simulink library "bcm"  (R2021b)
settings: Solver=VariableStepAuto  StartTime=0.0  StopTime=10.0  RelTol=1e-3
undefined symbols (not defined in the file or in its folder): ENUM_ANTITHEFT_ALARM, ENUM_ANTITHEFT_ARM, ENUM_ANTITHEFT_DISARM, ENUM_ANTITHEFT_WAIT, ENUM_GEARPOSNTOCAN_P, ENUM_PDKEYRAWLULOCK_INUNLOCK, ENUM_PDKEYRAWPS_INPS, ENUM_POWERSTA_ON, ENUM_POWERSTA_READY, ENUM_POWERSTA_STANDBY, FALSE, KBCM_ALMBrightnessDark_enum, KBCM_AmbBlue_enum, KBCM_AmbBreathT_ms, KBCM_AmbGreen_enum, KBCM_AmbRed_enum, KBCM_Antitheft_enum_ovrdflg, KBCM_Antitheft_enum_ovrdval, KBCM_APMDoorCtrlSta_flg_ovrdflg, KBCM_APMDoorCtrlSta_flg_ovrdval, KBCM_DelayTSW_flg, KBCM_DiagFLTC_mA, KBCM_DiagFMHT_s, KBCM_DiagFRTC_mA, KBCM_DiagRLTC_mA, KBCM_DiagRRTC_mA, KBCM_DrAPMRetryTimes_cnt, KBCM_DrOpenWdwOT_s, KBCM_DrOpenWdwReady_s, KBCM_ESSOffT_ms, KBCM_ESSOnT_ms, KBCM_IVIRstHoldT_ms, KBCM_IVIRstTriggerT_ms, KBCM_ONDelayT_ms, KBCM_ReDetectT_K, KBCM_RmLampKeep_min, KBCM_RmLpKeyInT_s, KBCM_RmLpKeyMissT_s, KBCM_SlpDebounceTime_s, KBCM_SPTGDetectT_sec, KBCM_SPTGLeave_flg, KBCM_SPTGLeftBound_cm, KBCM_SPTGLeftBoundOut_cm, KBCM_SPTGLowerBound_cm, KBCM_SPTGLowerBoundOut_cm, KBCM_SPTGRightBound_cm, KBCM_SPTGRightBoundOut_cm, KBCM_SPTGTOut_K, KBCM_SPTGUpperBound_cm, KBCM_SPTGUpperBoundOut_cm, KBCM_SPTGWaitDKC_sec, KBCM_TrunSWKeepTime3_s, KBCM_TrunSWKeepTime5_s, KBCM_TrunSWKeepTime7_s, KBCM_USSDis_cm, KBCM_USSFilterT_K, KBCM_WaitAPMPwr_K, KBCM_WdwManualDetT_s, MIN2SEC, TRUE ... (+1)
libraries: simulink x151, hcu_lib x5
(part 6 of 8)

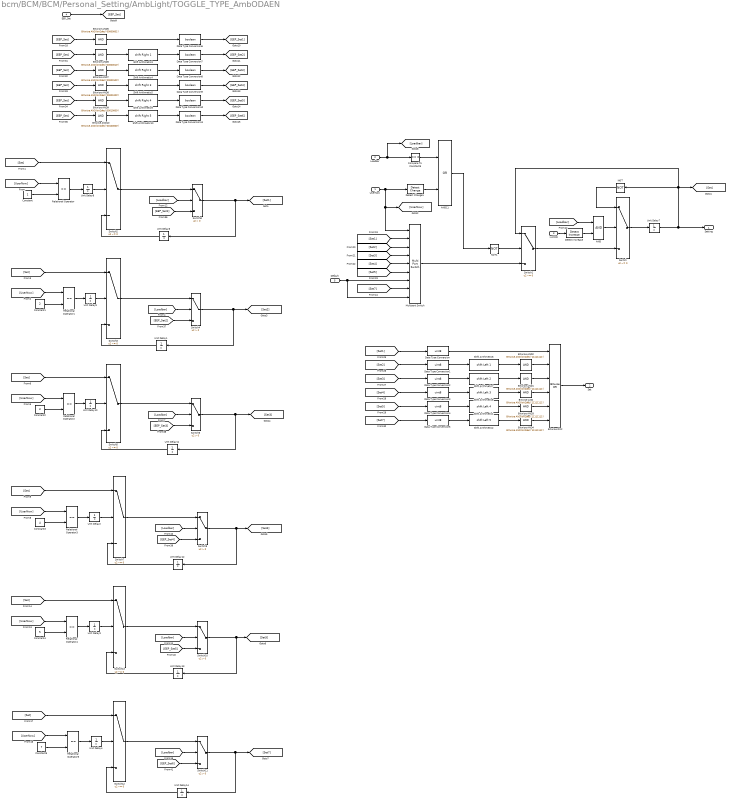
== system bcm/BCM/BCM/Personal_Setting/AmbLight/TOGGLE_TYPE_AmbODAEN ==
  UserNow : Inport
  Loadbar : Inport  Port=2
  iviCMD : Inport  Port=3
  EEP_Set : Inport  Port=4
  Default : Inport  Port=5
  AND : Logic  AllPortsSameDT=off  OutDataTypeStr=boolean
  AND11 : Logic  Operator=OR  AllPortsSameDT=off  OutDataTypeStr=boolean
  Bitwise AND{,1..4} (5 alike) : simulink/Logic and Bit Operations/Bitwise Operator  logicop=AND  UseBitMask=on  BitMask=bin2dec('11111111')  BitMaskRealWorld=Stored Integer
  Bitwise AND10 : simulink/Logic and Bit Operations/Bitwise Operator  logicop=AND  UseBitMask=on  BitMask=bin2dec('00100000')  BitMaskRealWorld=Stored Integer
  Bitwise AND5 : simulink/Logic and Bit Operations/Bitwise Operator  logicop=AND  UseBitMask=on  BitMask=bin2dec('00000001')  BitMaskRealWorld=Stored Integer
  Bitwise AND6 : simulink/Logic and Bit Operations/Bitwise Operator  logicop=AND  UseBitMask=on  BitMask=bin2dec('00000010')  BitMaskRealWorld=Stored Integer
  Bitwise AND7 : simulink/Logic and Bit Operations/Bitwise Operator  logicop=AND  UseBitMask=on  BitMask=bin2dec('00000100')  BitMaskRealWorld=Stored Integer
  Bitwise AND8 : simulink/Logic and Bit Operations/Bitwise Operator  logicop=AND  UseBitMask=on  BitMask=bin2dec('00001000')  BitMaskRealWorld=Stored Integer
  Bitwise AND9 : simulink/Logic and Bit Operations/Bitwise Operator  logicop=AND  UseBitMask=on  BitMask=bin2dec('00010000')  BitMaskRealWorld=Stored Integer
  Bitwise OR2 : simulink/Logic and Bit Operations/Bitwise Operator  logicop=OR  UseBitMask=off  NumInputPorts=6  BitMask=bin2dec('00000000000000000000')  BitMaskRealWorld=Stored Integer
  Compare To Constant5 : simulink/Logic and Bit Operations/Compare To Constant  relop===  const=0  OutDataTypeStr=boolean
  Constant : Constant  OutDataTypeStr=uint8
  Constant1 : Constant  Value=2  OutDataTypeStr=uint8
  Constant2 : Constant  Value=3  OutDataTypeStr=uint8
  Constant3 : Constant  Value=4  OutDataTypeStr=uint8
  Constant4 : Constant  Value=5  OutDataTypeStr=uint8
  Constant5 : Constant  Value=7  OutDataTypeStr=uint8
  Data Type Conversion{,1..5} (6 alike) : DataTypeConversion  OutDataTypeStr=uint8
  Data Type Conversion{6..11} (6 alike) : DataTypeConversion  OutDataTypeStr=boolean
  Detect Change1 : simulink/Logic and Bit Operations/Detect Change  vinit=0  OutDataTypeStr=boolean
  Detect Increase : simulink/Logic and Bit Operations/Detect Increase  vinit=0.0  OutDataTypeStr=boolean
  Multiport Switch : MultiPortSwitch  Inputs=7  DataPortForDefault=Additional data port  DiagnosticForDefault=None
  NOT : Logic  Operator=NOT  IconShape=distinctive  AllPortsSameDT=off  OutDataTypeStr=boolean
  NOT1 : Logic  Operator=NOT  IconShape=distinctive  AllPortsSameDT=off  OutDataTypeStr=boolean
  Relational Operator{,1..5} (6 alike) : RelationalOperator  Operator===  OutDataTypeStr=boolean  RndMeth=Simplest
  Shift Arithmetic1 : ArithShift  BitShiftNumber=4  BitShiftDirection=Left
  Shift Arithmetic10 : ArithShift  BitShiftNumber=5  BitShiftDirection=Right
  Shift Arithmetic2 : ArithShift  BitShiftNumber=5  BitShiftDirection=Left
  Shift Arithmetic3 : ArithShift  BitShiftNumber=1  BitShiftDirection=Right
  Shift Arithmetic4 : ArithShift  BitShiftNumber=2  BitShiftDirection=Right
  Shift Arithmetic5 : ArithShift  BitShiftNumber=3  BitShiftDirection=Right
  Shift Arithmetic6 : ArithShift  BitShiftNumber=1  BitShiftDirection=Left
  Shift Arithmetic7 : ArithShift  BitShiftNumber=2  BitShiftDirection=Left
  Shift Arithmetic8 : ArithShift  BitShiftNumber=3  BitShiftDirection=Left
  Shift Arithmetic9 : ArithShift  BitShiftNumber=4  BitShiftDirection=Right
  Switch{,1..3,5,7,12..13} (8 alike) : Switch  Criteria=u2 ~= 0
  Switch{4,6,8..11} (6 alike) : Switch  Criteria=u2 > Threshold
  Unit Delay{1..4,6..14} (13 alike) : UnitDelay  SampleTime=-1  HasFrameUpgradeWarning=on
  Setting : Outport
  Set : Outport  Port=2
  wires:
  [Loadbar] -> AND/1
  Detect Increase/1 -> AND/2
  AND/1 -> Switch/2
  Unit Delay14/1 -> Switch12/3
  Unit Delay4/1 -> Switch12/2
  Unit Delay13/1 -> Switch13/3
  Unit Delay3/1 -> Switch13/2
  Unit Delay12/1 -> Switch7/3
  Unit Delay2/1 -> Switch7/2
  Unit Delay11/1 -> Switch5/3
  Unit Delay10/1 -> Switch5/2
  Unit Delay9/1 -> Switch3/2
  Unit Delay8/1 -> Switch2/2
  Unit Delay1/1 -> Switch3/3
  Unit Delay6/1 -> Switch2/3
  Relational Operator1/1 -> Unit Delay9/1
  Relational Operator/1 -> Unit Delay8/1
  [EEP_Set6] -> Switch11/3
  [EEP_Set5] -> Switch10/3
  [EEP_Set4] -> Switch9/3
  [EEP_Set3] -> Switch6/3
  [EEP_Set2] -> Switch4/3
  [EEP_Set1] -> Switch8/3
  Data Type Conversion11/1 -> [EEP_Set6]
  Data Type Conversion10/1 -> [EEP_Set5]
  Data Type Conversion9/1 -> [EEP_Set4]
  Data Type Conversion8/1 -> [EEP_Set3]
  Data Type Conversion7/1 -> [EEP_Set2]
  Data Type Conversion6/1 -> [EEP_Set1]
  [EEP_Set] -> Bitwise AND10/1
  [EEP_Set] -> Bitwise AND9/1
  [EEP_Set] -> Bitwise AND8/1
  [EEP_Set] -> Bitwise AND7/1
  [EEP_Set] -> Bitwise AND6/1
  [EEP_Set] -> Bitwise AND5/1
  EEP_Set/1 -> [EEP_Set]
  Shift Arithmetic5/1 -> Data Type Conversion9/1
  Shift Arithmetic9/1 -> Data Type Conversion10/1
  Bitwise AND7/1 -> Shift Arithmetic4/1
  Shift Arithmetic3/1 -> Data Type Conversion7/1
  Bitwise AND5/1 -> Data Type Conversion6/1
  Shift Arithmetic10/1 -> Data Type Conversion11/1
  Shift Arithmetic4/1 -> Data Type Conversion8/1
  Bitwise AND10/1 -> Shift Arithmetic10/1
  Bitwise AND9/1 -> Shift Arithmetic9/1
  Bitwise AND6/1 -> Shift Arithmetic3/1
  Bitwise AND8/1 -> Shift Arithmetic5/1
  Bitwise OR2/1 -> Set/1
  [Set3] -> Data Type Conversion2/1
  Bitwise AND4/1 -> Bitwise OR2/6
  Data Type Conversion1/1 -> Shift Arithmetic6/1
  Bitwise AND/1 -> Bitwise OR2/4
  [Set5] -> Data Type Conversion4/1
  [Set1] -> Data Type Conversion/1
  Data Type Conversion3/1 -> Shift Arithmetic8/1
  [Set2] -> Data Type Conversion1/1
  Data Type Conversion/1 -> Bitwise OR2/1
  [Set7] -> Data Type Conversion5/1
  Shift Arithmetic1/1 -> Bitwise AND3/1
  Shift Arithmetic7/1 -> Bitwise AND1/1
  Data Type Conversion4/1 -> Shift Arithmetic1/1
  Shift Arithmetic6/1 -> Bitwise AND2/1
  Bitwise AND2/1 -> Bitwise OR2/2
  Bitwise AND1/1 -> Bitwise OR2/3
  Bitwise AND3/1 -> Bitwise OR2/5
  Shift Arithmetic2/1 -> Bitwise AND4/1
  Shift Arithmetic8/1 -> Bitwise AND/1
  [Set4] -> Data Type Conversion3/1
  Data Type Conversion5/1 -> Shift Arithmetic2/1
  Data Type Conversion2/1 -> Shift Arithmetic7/1
  Relational Operator5/1 -> Unit Delay4/1
  Relational Operator4/1 -> Unit Delay3/1
  Relational Operator3/1 -> Unit Delay2/1
  Relational Operator2/1 -> Unit Delay10/1
  Unit Delay7/1 -> Switch1/1, [Set], NOT/1, Setting/1
  Switch11/1 -> Unit Delay14/1, [Set7]
  Switch12/1 -> Switch11/1
  Switch10/1 -> Unit Delay13/1, [Set5]
  Switch9/1 -> Unit Delay12/1, [Set4]
  Switch7/1 -> Switch9/1
  Switch5/1 -> Switch6/1
  Switch6/1 -> Unit Delay11/1, [Set3]
  Switch4/1 -> Unit Delay1/1, [Set2]
  Switch3/1 -> Switch4/1
  Switch2/1 -> Switch8/1
  Switch8/1 -> Unit Delay6/1, [Set1]
  Switch/1 -> Unit Delay7/1
  AND11/1 -> NOT1/1
  Compare To Constant5/1 -> AND11/1
  Constant4/1 -> Relational Operator4/2
  [Loadbar] -> Switch8/2
  [Set] -> Switch5/1
  [Loadbar] -> Switch6/2
  [Set] -> Switch7/1
  Constant1/1 -> Relational Operator1/2
  [UserNow] -> Relational Operator4/1
  [Set] -> Switch2/1
  Constant3/1 -> Relational Operator3/2
  [UserNow] -> Relational Operator3/1
  [UserNow] -> Relational Operator2/1
  [Loadbar] -> Switch9/2
  Constant/1 -> Relational Operator/2
  [Set] -> Switch3/1
  [Loadbar] -> Switch11/2
  Constant2/1 -> Relational Operator2/2
  [Loadbar] -> Switch10/2
  [UserNow] -> Relational Operator1/1
  [UserNow] -> Relational Operator/1
  Constant5/1 -> Relational Operator5/2
  [UserNow] -> Relational Operator5/1
  [Set] -> Switch12/1
  [Loadbar] -> Switch4/2
  [Set] -> Switch13/1
  iviCMD/1 -> Detect Increase/1
  NOT/1 -> Switch/1
  UserNow/1 -> Detect Change1/1, [UserNow], Multiport Switch/1
  Switch1/1 -> Switch/3
  Loadbar/1 -> Compare To Constant5/1, [Loadbar]
  Multiport Switch/1 -> Switch1/3
  Detect Change1/1 -> AND11/2
  Switch13/1 -> Switch10/1
  NOT1/1 -> Switch1/2
  [Set1] -> Multiport Switch/2
  [Set2] -> Multiport Switch/3
  [Set3] -> Multiport Switch/4
  [Set4] -> Multiport Switch/5
  [Set5] -> Multiport Switch/6
  [Set7] -> Multiport Switch/8
  Default/1 -> Multiport Switch/9, Multiport Switch/7

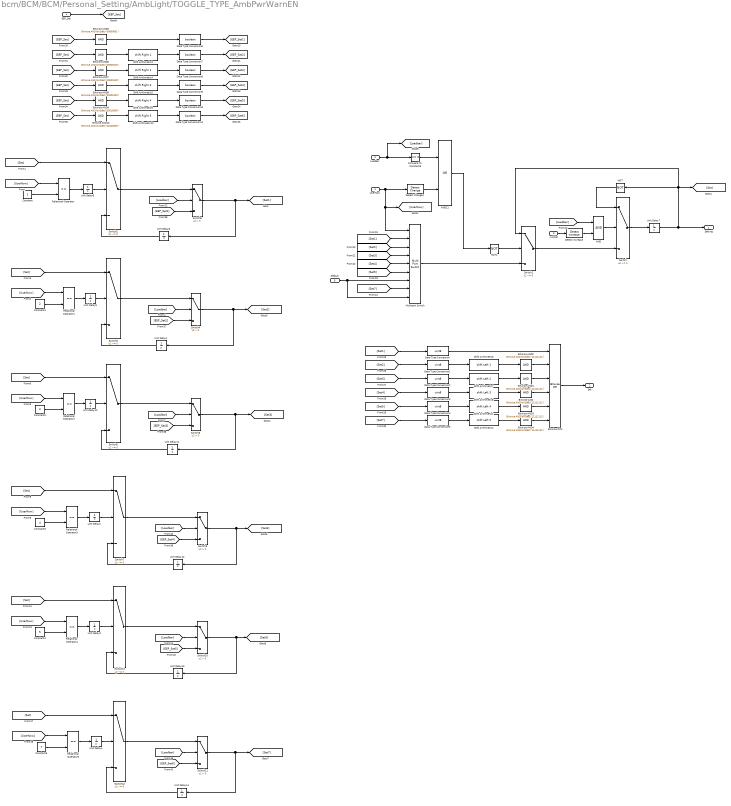
== system bcm/BCM/BCM/Personal_Setting/AmbLight/TOGGLE_TYPE_AmbPwrWarnEN ==
  UserNow : Inport
  Loadbar : Inport  Port=2
  iviCMD : Inport  Port=3
  EEP_Set : Inport  Port=4
  Default : Inport  Port=5
  AND : Logic  AllPortsSameDT=off  OutDataTypeStr=boolean
  AND11 : Logic  Operator=OR  AllPortsSameDT=off  OutDataTypeStr=boolean
  Bitwise AND{,1..4} (5 alike) : simulink/Logic and Bit Operations/Bitwise Operator  logicop=AND  UseBitMask=on  BitMask=bin2dec('11111111')  BitMaskRealWorld=Stored Integer
  Bitwise AND10 : simulink/Logic and Bit Operations/Bitwise Operator  logicop=AND  UseBitMask=on  BitMask=bin2dec('00100000')  BitMaskRealWorld=Stored Integer
  Bitwise AND5 : simulink/Logic and Bit Operations/Bitwise Operator  logicop=AND  UseBitMask=on  BitMask=bin2dec('00000001')  BitMaskRealWorld=Stored Integer
  Bitwise AND6 : simulink/Logic and Bit Operations/Bitwise Operator  logicop=AND  UseBitMask=on  BitMask=bin2dec('00000010')  BitMaskRealWorld=Stored Integer
  Bitwise AND7 : simulink/Logic and Bit Operations/Bitwise Operator  logicop=AND  UseBitMask=on  BitMask=bin2dec('00000100')  BitMaskRealWorld=Stored Integer
  Bitwise AND8 : simulink/Logic and Bit Operations/Bitwise Operator  logicop=AND  UseBitMask=on  BitMask=bin2dec('00001000')  BitMaskRealWorld=Stored Integer
  Bitwise AND9 : simulink/Logic and Bit Operations/Bitwise Operator  logicop=AND  UseBitMask=on  BitMask=bin2dec('00010000')  BitMaskRealWorld=Stored Integer
  Bitwise OR2 : simulink/Logic and Bit Operations/Bitwise Operator  logicop=OR  UseBitMask=off  NumInputPorts=6  BitMask=bin2dec('00000000000000000000')  BitMaskRealWorld=Stored Integer
  Compare To Constant5 : simulink/Logic and Bit Operations/Compare To Constant  relop===  const=0  OutDataTypeStr=boolean
  Constant : Constant  OutDataTypeStr=uint8
  Constant1 : Constant  Value=2  OutDataTypeStr=uint8
  Constant2 : Constant  Value=3  OutDataTypeStr=uint8
  Constant3 : Constant  Value=4  OutDataTypeStr=uint8
  Constant4 : Constant  Value=5  OutDataTypeStr=uint8
  Constant5 : Constant  Value=7  OutDataTypeStr=uint8
  Data Type Conversion{,1..5} (6 alike) : DataTypeConversion  OutDataTypeStr=uint8
  Data Type Conversion{6..11} (6 alike) : DataTypeConversion  OutDataTypeStr=boolean
  Detect Change1 : simulink/Logic and Bit Operations/Detect Change  vinit=0  OutDataTypeStr=boolean
  Detect Increase : simulink/Logic and Bit Operations/Detect Increase  vinit=0.0  OutDataTypeStr=boolean
  Multiport Switch : MultiPortSwitch  Inputs=7  DataPortForDefault=Additional data port  DiagnosticForDefault=None
  NOT : Logic  Operator=NOT  IconShape=distinctive  AllPortsSameDT=off  OutDataTypeStr=boolean
  NOT1 : Logic  Operator=NOT  IconShape=distinctive  AllPortsSameDT=off  OutDataTypeStr=boolean
  Relational Operator{,1..5} (6 alike) : RelationalOperator  Operator===  OutDataTypeStr=boolean  RndMeth=Simplest
  Shift Arithmetic1 : ArithShift  BitShiftNumber=4  BitShiftDirection=Left
  Shift Arithmetic10 : ArithShift  BitShiftNumber=5  BitShiftDirection=Right
  Shift Arithmetic2 : ArithShift  BitShiftNumber=5  BitShiftDirection=Left
  Shift Arithmetic3 : ArithShift  BitShiftNumber=1  BitShiftDirection=Right
  Shift Arithmetic4 : ArithShift  BitShiftNumber=2  BitShiftDirection=Right
  Shift Arithmetic5 : ArithShift  BitShiftNumber=3  BitShiftDirection=Right
  Shift Arithmetic6 : ArithShift  BitShiftNumber=1  BitShiftDirection=Left
  Shift Arithmetic7 : ArithShift  BitShiftNumber=2  BitShiftDirection=Left
  Shift Arithmetic8 : ArithShift  BitShiftNumber=3  BitShiftDirection=Left
  Shift Arithmetic9 : ArithShift  BitShiftNumber=4  BitShiftDirection=Right
  Switch{,1..3,5,7,12..13} (8 alike) : Switch  Criteria=u2 ~= 0
  Switch{4,6,8..11} (6 alike) : Switch  Criteria=u2 > Threshold
  Unit Delay{1..4,6..14} (13 alike) : UnitDelay  SampleTime=-1  HasFrameUpgradeWarning=on
  Setting : Outport
  Set : Outport  Port=2
  wires:
  Default/1 -> Multiport Switch/7, Multiport Switch/9
  [Set7] -> Multiport Switch/8
  [Set5] -> Multiport Switch/6
  [Set4] -> Multiport Switch/5
  [Set3] -> Multiport Switch/4
  [Set2] -> Multiport Switch/3
  [Set1] -> Multiport Switch/2
  NOT1/1 -> Switch1/2
  Switch13/1 -> Switch10/1
  Detect Change1/1 -> AND11/2
  Multiport Switch/1 -> Switch1/3
  Loadbar/1 -> [Loadbar], Compare To Constant5/1
  Switch1/1 -> Switch/3
  UserNow/1 -> Multiport Switch/1, [UserNow], Detect Change1/1
  NOT/1 -> Switch/1
  iviCMD/1 -> Detect Increase/1
  [Set] -> Switch13/1
  [Loadbar] -> Switch4/2
  [Set] -> Switch12/1
  [UserNow] -> Relational Operator5/1
  Constant5/1 -> Relational Operator5/2
  [UserNow] -> Relational Operator/1
  [UserNow] -> Relational Operator1/1
  [Loadbar] -> Switch10/2
  Constant2/1 -> Relational Operator2/2
  [Loadbar] -> Switch11/2
  [Set] -> Switch3/1
  Constant/1 -> Relational Operator/2
  [Loadbar] -> Switch9/2
  [UserNow] -> Relational Operator2/1
  [UserNow] -> Relational Operator3/1
  Constant3/1 -> Relational Operator3/2
  [Set] -> Switch2/1
  [UserNow] -> Relational Operator4/1
  Constant1/1 -> Relational Operator1/2
  [Set] -> Switch7/1
  [Loadbar] -> Switch6/2
  [Set] -> Switch5/1
  [Loadbar] -> Switch8/2
  Constant4/1 -> Relational Operator4/2
  Compare To Constant5/1 -> AND11/1
  AND11/1 -> NOT1/1
  Switch/1 -> Unit Delay7/1
  Switch8/1 -> [Set1], Unit Delay6/1
  Switch2/1 -> Switch8/1
  Switch3/1 -> Switch4/1
  Switch4/1 -> [Set2], Unit Delay1/1
  Switch6/1 -> [Set3], Unit Delay11/1
  Switch5/1 -> Switch6/1
  Switch7/1 -> Switch9/1
  Switch9/1 -> [Set4], Unit Delay12/1
  Switch10/1 -> [Set5], Unit Delay13/1
  Switch12/1 -> Switch11/1
  Switch11/1 -> [Set7], Unit Delay14/1
  Unit Delay7/1 -> Setting/1, NOT/1, [Set], Switch1/1
  Relational Operator2/1 -> Unit Delay10/1
  Relational Operator3/1 -> Unit Delay2/1
  Relational Operator4/1 -> Unit Delay3/1
  Relational Operator5/1 -> Unit Delay4/1
  Data Type Conversion2/1 -> Shift Arithmetic7/1
  Data Type Conversion5/1 -> Shift Arithmetic2/1
  [Set4] -> Data Type Conversion3/1
  Shift Arithmetic8/1 -> Bitwise AND/1
  Shift Arithmetic2/1 -> Bitwise AND4/1
  Bitwise AND3/1 -> Bitwise OR2/5
  Bitwise AND1/1 -> Bitwise OR2/3
  Bitwise AND2/1 -> Bitwise OR2/2
  Shift Arithmetic6/1 -> Bitwise AND2/1
  Data Type Conversion4/1 -> Shift Arithmetic1/1
  Shift Arithmetic7/1 -> Bitwise AND1/1
  Shift Arithmetic1/1 -> Bitwise AND3/1
  [Set7] -> Data Type Conversion5/1
  Data Type Conversion/1 -> Bitwise OR2/1
  [Set2] -> Data Type Conversion1/1
  Data Type Conversion3/1 -> Shift Arithmetic8/1
  [Set1] -> Data Type Conversion/1
  [Set5] -> Data Type Conversion4/1
  Bitwise AND/1 -> Bitwise OR2/4
  Data Type Conversion1/1 -> Shift Arithmetic6/1
  Bitwise AND4/1 -> Bitwise OR2/6
  [Set3] -> Data Type Conversion2/1
  Bitwise OR2/1 -> Set/1
  Bitwise AND8/1 -> Shift Arithmetic5/1
  Bitwise AND6/1 -> Shift Arithmetic3/1
  Bitwise AND9/1 -> Shift Arithmetic9/1
  Bitwise AND10/1 -> Shift Arithmetic10/1
  Shift Arithmetic4/1 -> Data Type Conversion8/1
  Shift Arithmetic10/1 -> Data Type Conversion11/1
  Bitwise AND5/1 -> Data Type Conversion6/1
  Shift Arithmetic3/1 -> Data Type Conversion7/1
  Bitwise AND7/1 -> Shift Arithmetic4/1
  Shift Arithmetic9/1 -> Data Type Conversion10/1
  Shift Arithmetic5/1 -> Data Type Conversion9/1
  EEP_Set/1 -> [EEP_Set]
  [EEP_Set] -> Bitwise AND5/1
  [EEP_Set] -> Bitwise AND6/1
  [EEP_Set] -> Bitwise AND7/1
  [EEP_Set] -> Bitwise AND8/1
  [EEP_Set] -> Bitwise AND9/1
  [EEP_Set] -> Bitwise AND10/1
  Data Type Conversion6/1 -> [EEP_Set1]
  Data Type Conversion7/1 -> [EEP_Set2]
  Data Type Conversion8/1 -> [EEP_Set3]
  Data Type Conversion9/1 -> [EEP_Set4]
  Data Type Conversion10/1 -> [EEP_Set5]
  Data Type Conversion11/1 -> [EEP_Set6]
  [EEP_Set1] -> Switch8/3
  [EEP_Set2] -> Switch4/3
  [EEP_Set3] -> Switch6/3
  [EEP_Set4] -> Switch9/3
  [EEP_Set5] -> Switch10/3
  [EEP_Set6] -> Switch11/3
  Relational Operator/1 -> Unit Delay8/1
  Relational Operator1/1 -> Unit Delay9/1
  Unit Delay6/1 -> Switch2/3
  Unit Delay1/1 -> Switch3/3
  Unit Delay8/1 -> Switch2/2
  Unit Delay9/1 -> Switch3/2
  Unit Delay10/1 -> Switch5/2
  Unit Delay11/1 -> Switch5/3
  Unit Delay2/1 -> Switch7/2
  Unit Delay12/1 -> Switch7/3
  Unit Delay3/1 -> Switch13/2
  Unit Delay13/1 -> Switch13/3
  Unit Delay4/1 -> Switch12/2
  Unit Delay14/1 -> Switch12/3
  AND/1 -> Switch/2
  Detect Increase/1 -> AND/2
  [Loadbar] -> AND/1

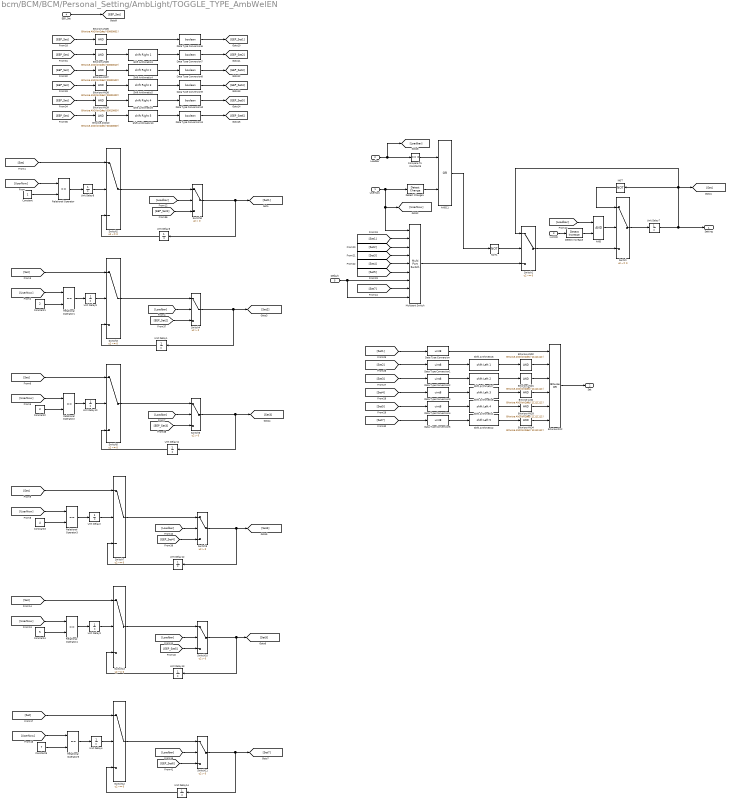
== system bcm/BCM/BCM/Personal_Setting/AmbLight/TOGGLE_TYPE_AmbWelEN ==
  UserNow : Inport
  Loadbar : Inport  Port=2
  iviCMD : Inport  Port=3
  EEP_Set : Inport  Port=4
  Default : Inport  Port=5
  AND : Logic  AllPortsSameDT=off  OutDataTypeStr=boolean
  AND11 : Logic  Operator=OR  AllPortsSameDT=off  OutDataTypeStr=boolean
  Bitwise AND{,1..4} (5 alike) : simulink/Logic and Bit Operations/Bitwise Operator  logicop=AND  UseBitMask=on  BitMask=bin2dec('11111111')  BitMaskRealWorld=Stored Integer
  Bitwise AND10 : simulink/Logic and Bit Operations/Bitwise Operator  logicop=AND  UseBitMask=on  BitMask=bin2dec('00100000')  BitMaskRealWorld=Stored Integer
  Bitwise AND5 : simulink/Logic and Bit Operations/Bitwise Operator  logicop=AND  UseBitMask=on  BitMask=bin2dec('00000001')  BitMaskRealWorld=Stored Integer
  Bitwise AND6 : simulink/Logic and Bit Operations/Bitwise Operator  logicop=AND  UseBitMask=on  BitMask=bin2dec('00000010')  BitMaskRealWorld=Stored Integer
  Bitwise AND7 : simulink/Logic and Bit Operations/Bitwise Operator  logicop=AND  UseBitMask=on  BitMask=bin2dec('00000100')  BitMaskRealWorld=Stored Integer
  Bitwise AND8 : simulink/Logic and Bit Operations/Bitwise Operator  logicop=AND  UseBitMask=on  BitMask=bin2dec('00001000')  BitMaskRealWorld=Stored Integer
  Bitwise AND9 : simulink/Logic and Bit Operations/Bitwise Operator  logicop=AND  UseBitMask=on  BitMask=bin2dec('00010000')  BitMaskRealWorld=Stored Integer
  Bitwise OR2 : simulink/Logic and Bit Operations/Bitwise Operator  logicop=OR  UseBitMask=off  NumInputPorts=6  BitMask=bin2dec('00000000000000000000')  BitMaskRealWorld=Stored Integer
  Compare To Constant5 : simulink/Logic and Bit Operations/Compare To Constant  relop===  const=0  OutDataTypeStr=boolean
  Constant : Constant  OutDataTypeStr=uint8
  Constant1 : Constant  Value=2  OutDataTypeStr=uint8
  Constant2 : Constant  Value=3  OutDataTypeStr=uint8
  Constant3 : Constant  Value=4  OutDataTypeStr=uint8
  Constant4 : Constant  Value=5  OutDataTypeStr=uint8
  Constant5 : Constant  Value=7  OutDataTypeStr=uint8
  Data Type Conversion{,1..5} (6 alike) : DataTypeConversion  OutDataTypeStr=uint8
  Data Type Conversion{6..11} (6 alike) : DataTypeConversion  OutDataTypeStr=boolean
  Detect Change1 : simulink/Logic and Bit Operations/Detect Change  vinit=0  OutDataTypeStr=boolean
  Detect Increase : simulink/Logic and Bit Operations/Detect Increase  vinit=0.0  OutDataTypeStr=boolean
  Multiport Switch : MultiPortSwitch  Inputs=7  DataPortForDefault=Additional data port  DiagnosticForDefault=None
  NOT : Logic  Operator=NOT  IconShape=distinctive  AllPortsSameDT=off  OutDataTypeStr=boolean
  NOT1 : Logic  Operator=NOT  IconShape=distinctive  AllPortsSameDT=off  OutDataTypeStr=boolean
  Relational Operator{,1..5} (6 alike) : RelationalOperator  Operator===  OutDataTypeStr=boolean  RndMeth=Simplest
  Shift Arithmetic1 : ArithShift  BitShiftNumber=4  BitShiftDirection=Left
  Shift Arithmetic10 : ArithShift  BitShiftNumber=5  BitShiftDirection=Right
  Shift Arithmetic2 : ArithShift  BitShiftNumber=5  BitShiftDirection=Left
  Shift Arithmetic3 : ArithShift  BitShiftNumber=1  BitShiftDirection=Right
  Shift Arithmetic4 : ArithShift  BitShiftNumber=2  BitShiftDirection=Right
  Shift Arithmetic5 : ArithShift  BitShiftNumber=3  BitShiftDirection=Right
  Shift Arithmetic6 : ArithShift  BitShiftNumber=1  BitShiftDirection=Left
  Shift Arithmetic7 : ArithShift  BitShiftNumber=2  BitShiftDirection=Left
  Shift Arithmetic8 : ArithShift  BitShiftNumber=3  BitShiftDirection=Left
  Shift Arithmetic9 : ArithShift  BitShiftNumber=4  BitShiftDirection=Right
  Switch{,1..3,5,7,12..13} (8 alike) : Switch  Criteria=u2 ~= 0
  Switch{4,6,8..11} (6 alike) : Switch  Criteria=u2 > Threshold
  Unit Delay{1..4,6..14} (13 alike) : UnitDelay  SampleTime=-1  HasFrameUpgradeWarning=on
  Setting : Outport
  Set : Outport  Port=2
  wires:
  [Loadbar] -> AND/1
  Detect Increase/1 -> AND/2
  AND/1 -> Switch/2
  Unit Delay14/1 -> Switch12/3
  Unit Delay4/1 -> Switch12/2
  Unit Delay13/1 -> Switch13/3
  Unit Delay3/1 -> Switch13/2
  Unit Delay12/1 -> Switch7/3
  Unit Delay2/1 -> Switch7/2
  Unit Delay11/1 -> Switch5/3
  Unit Delay10/1 -> Switch5/2
  Unit Delay9/1 -> Switch3/2
  Unit Delay8/1 -> Switch2/2
  Unit Delay1/1 -> Switch3/3
  Unit Delay6/1 -> Switch2/3
  Relational Operator1/1 -> Unit Delay9/1
  Relational Operator/1 -> Unit Delay8/1
  [EEP_Set6] -> Switch11/3
  [EEP_Set5] -> Switch10/3
  [EEP_Set4] -> Switch9/3
  [EEP_Set3] -> Switch6/3
  [EEP_Set2] -> Switch4/3
  [EEP_Set1] -> Switch8/3
  Data Type Conversion11/1 -> [EEP_Set6]
  Data Type Conversion10/1 -> [EEP_Set5]
  Data Type Conversion9/1 -> [EEP_Set4]
  Data Type Conversion8/1 -> [EEP_Set3]
  Data Type Conversion7/1 -> [EEP_Set2]
  Data Type Conversion6/1 -> [EEP_Set1]
  [EEP_Set] -> Bitwise AND10/1
  [EEP_Set] -> Bitwise AND9/1
  [EEP_Set] -> Bitwise AND8/1
  [EEP_Set] -> Bitwise AND7/1
  [EEP_Set] -> Bitwise AND6/1
  [EEP_Set] -> Bitwise AND5/1
  EEP_Set/1 -> [EEP_Set]
  Shift Arithmetic5/1 -> Data Type Conversion9/1
  Shift Arithmetic9/1 -> Data Type Conversion10/1
  Bitwise AND7/1 -> Shift Arithmetic4/1
  Shift Arithmetic3/1 -> Data Type Conversion7/1
  Bitwise AND5/1 -> Data Type Conversion6/1
  Shift Arithmetic10/1 -> Data Type Conversion11/1
  Shift Arithmetic4/1 -> Data Type Conversion8/1
  Bitwise AND10/1 -> Shift Arithmetic10/1
  Bitwise AND9/1 -> Shift Arithmetic9/1
  Bitwise AND6/1 -> Shift Arithmetic3/1
  Bitwise AND8/1 -> Shift Arithmetic5/1
  Bitwise OR2/1 -> Set/1
  [Set3] -> Data Type Conversion2/1
  Bitwise AND4/1 -> Bitwise OR2/6
  Data Type Conversion1/1 -> Shift Arithmetic6/1
  Bitwise AND/1 -> Bitwise OR2/4
  [Set5] -> Data Type Conversion4/1
  [Set1] -> Data Type Conversion/1
  Data Type Conversion3/1 -> Shift Arithmetic8/1
  [Set2] -> Data Type Conversion1/1
  Data Type Conversion/1 -> Bitwise OR2/1
  [Set7] -> Data Type Conversion5/1
  Shift Arithmetic1/1 -> Bitwise AND3/1
  Shift Arithmetic7/1 -> Bitwise AND1/1
  Data Type Conversion4/1 -> Shift Arithmetic1/1
  Shift Arithmetic6/1 -> Bitwise AND2/1
  Bitwise AND2/1 -> Bitwise OR2/2
  Bitwise AND1/1 -> Bitwise OR2/3
  Bitwise AND3/1 -> Bitwise OR2/5
  Shift Arithmetic2/1 -> Bitwise AND4/1
  Shift Arithmetic8/1 -> Bitwise AND/1
  [Set4] -> Data Type Conversion3/1
  Data Type Conversion5/1 -> Shift Arithmetic2/1
  Data Type Conversion2/1 -> Shift Arithmetic7/1
  Relational Operator5/1 -> Unit Delay4/1
  Relational Operator4/1 -> Unit Delay3/1
  Relational Operator3/1 -> Unit Delay2/1
  Relational Operator2/1 -> Unit Delay10/1
  Unit Delay7/1 -> Switch1/1, [Set], NOT/1, Setting/1
  Switch11/1 -> Unit Delay14/1, [Set7]
  Switch12/1 -> Switch11/1
  Switch10/1 -> Unit Delay13/1, [Set5]
  Switch9/1 -> Unit Delay12/1, [Set4]
  Switch7/1 -> Switch9/1
  Switch5/1 -> Switch6/1
  Switch6/1 -> Unit Delay11/1, [Set3]
  Switch4/1 -> Unit Delay1/1, [Set2]
  Switch3/1 -> Switch4/1
  Switch2/1 -> Switch8/1
  Switch8/1 -> Unit Delay6/1, [Set1]
  Switch/1 -> Unit Delay7/1
  AND11/1 -> NOT1/1
  Compare To Constant5/1 -> AND11/1
  Constant4/1 -> Relational Operator4/2
  [Loadbar] -> Switch8/2
  [Set] -> Switch5/1
  [Loadbar] -> Switch6/2
  [Set] -> Switch7/1
  Constant1/1 -> Relational Operator1/2
  [UserNow] -> Relational Operator4/1
  [Set] -> Switch2/1
  Constant3/1 -> Relational Operator3/2
  [UserNow] -> Relational Operator3/1
  [UserNow] -> Relational Operator2/1
  [Loadbar] -> Switch9/2
  Constant/1 -> Relational Operator/2
  [Set] -> Switch3/1
  [Loadbar] -> Switch11/2
  Constant2/1 -> Relational Operator2/2
  [Loadbar] -> Switch10/2
  [UserNow] -> Relational Operator1/1
  [UserNow] -> Relational Operator/1
  Constant5/1 -> Relational Operator5/2
  [UserNow] -> Relational Operator5/1
  [Set] -> Switch12/1
  [Loadbar] -> Switch4/2
  [Set] -> Switch13/1
  iviCMD/1 -> Detect Increase/1
  NOT/1 -> Switch/1
  UserNow/1 -> Detect Change1/1, [UserNow], Multiport Switch/1
  Switch1/1 -> Switch/3
  Loadbar/1 -> Compare To Constant5/1, [Loadbar]
  Multiport Switch/1 -> Switch1/3
  Detect Change1/1 -> AND11/2
  Switch13/1 -> Switch10/1
  NOT1/1 -> Switch1/2
  [Set1] -> Multiport Switch/2
  [Set2] -> Multiport Switch/3
  [Set3] -> Multiport Switch/4
  [Set4] -> Multiport Switch/5
  [Set5] -> Multiport Switch/6
  [Set7] -> Multiport Switch/8
  Default/1 -> Multiport Switch/9, Multiport Switch/7

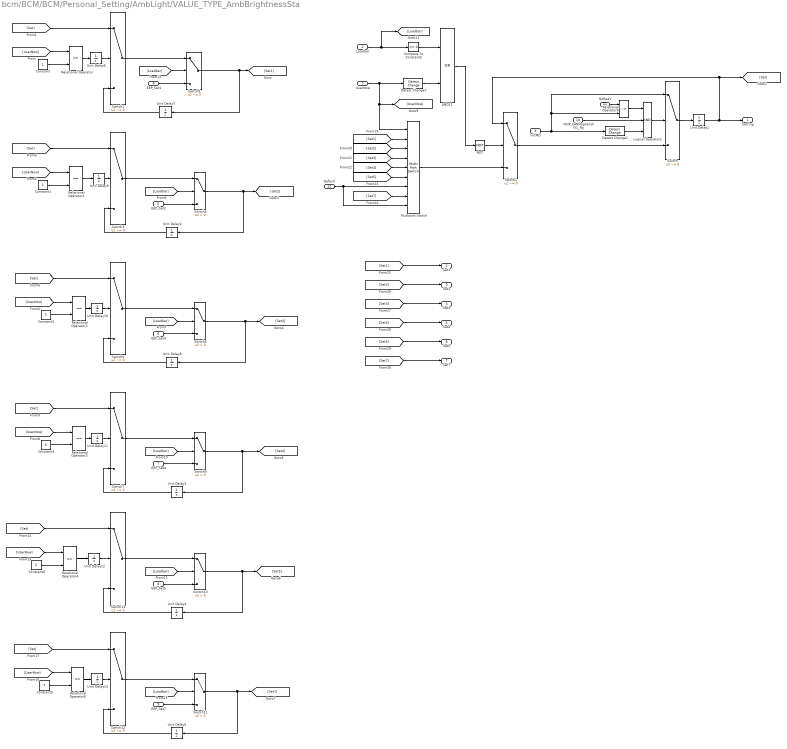
== system bcm/BCM/BCM/Personal_Setting/AmbLight/VALUE_TYPE_AmbBrightnessSta ==
  UserNow : Inport
  Loadbar : Inport  Port=2
  iviCMD : Inport  Port=3
  EEP_Set1 : Inport  Port=4
  EEP_Set2 : Inport  Port=5
  EEP_Set3 : Inport  Port=6
  EEP_Set4 : Inport  Port=7
  EEP_Set5 : Inport  Port=8
  EEP_Set7 : Inport  Port=9
  VINP_CANMsgValidIVI1_flg : Inport  Port=10
  NoReqV : Inport  Port=11
  Default : Inport  Port=12
  AND11 : Logic  Operator=OR  AllPortsSameDT=off  OutDataTypeStr=boolean
  Compare To Constant5 : simulink/Logic and Bit Operations/Compare To Constant  relop===  const=0  OutDataTypeStr=boolean
  Constant : Constant  OutDataTypeStr=uint8
  Constant1 : Constant  Value=2  OutDataTypeStr=uint8
  Constant2 : Constant  Value=3  OutDataTypeStr=uint8
  Constant3 : Constant  Value=4  OutDataTypeStr=uint8
  Constant4 : Constant  Value=5  OutDataTypeStr=uint8
  Constant5 : Constant  Value=7  OutDataTypeStr=uint8
  Detect Change1 : simulink/Logic and Bit Operations/Detect Change  vinit=0  OutDataTypeStr=boolean
  Detect Change7 : simulink/Logic and Bit Operations/Detect Change  vinit=0  OutDataTypeStr=boolean
  Logical Operator1 : Logic  Inputs=3  AllPortsSameDT=off  OutDataTypeStr=boolean
  Multiport Switch : MultiPortSwitch  Inputs=7  DataPortForDefault=Additional data port  DiagnosticForDefault=None
  NOT : Logic  Operator=NOT  IconShape=distinctive  AllPortsSameDT=off  OutDataTypeStr=boolean
  Relational Operator{,1..5} (6 alike) : RelationalOperator  Operator===  OutDataTypeStr=boolean  RndMeth=Simplest
  Relational Operator6 : RelationalOperator  Operator=~=  OutDataTypeStr=boolean  RndMeth=Simplest
  Switch{,1..3,5,7..8,12..13} (9 alike) : Switch  Criteria=u2 ~= 0
  Switch{4,6,9..11} (5 alike) : Switch  Criteria=u2 > Threshold
  Unit Delay{1..13} (13 alike) : UnitDelay  SampleTime=-1  HasFrameUpgradeWarning=on
  Setting : Outport
  Set1 : Outport  Port=2
  Set2 : Outport  Port=3
  Set3 : Outport  Port=4
  Set4 : Outport  Port=5
  Set5 : Outport  Port=6
  Set7 : Outport  Port=7
  wires:
  VINP_CANMsgValidIVI1_flg/1 -> Logical Operator1/2
  Unit Delay13/1 -> Switch12/2
  Unit Delay12/1 -> Switch13/2
  Unit Delay11/1 -> Switch7/2
  Unit Delay10/1 -> Switch5/2
  Unit Delay9/1 -> Switch3/2
  Unit Delay6/1 -> Switch2/2
  Unit Delay5/1 -> Switch12/3
  Unit Delay4/1 -> Switch13/3
  Unit Delay3/1 -> Switch7/3
  Unit Delay8/1 -> Switch5/3
  Unit Delay2/1 -> Switch3/3
  Unit Delay7/1 -> Switch2/3
  Unit Delay1/1 -> Setting/1, [Set], Switch1/1
  Switch/1 -> Unit Delay1/1
  Loadbar/1 -> Compare To Constant5/1, [Loadbar]
  UserNow/1 -> Detect Change7/1, [UserNow], Multiport Switch/1
  Compare To Constant5/1 -> AND11/1
  AND11/1 -> NOT/1
  [Set7] -> Set7/1
  [Set5] -> Set5/1
  [Set4] -> Set4/1
  [Set3] -> Set3/1
  [Set2] -> Set2/1
  [Set1] -> Set1/1
  Switch1/1 -> Switch/3
  Logical Operator1/1 -> Switch/2
  Multiport Switch/1 -> Switch1/3
  iviCMD/1 -> Relational Operator6/2, Switch/1, Detect Change1/1
  Detect Change1/1 -> Logical Operator1/3
  Relational Operator6/1 -> Logical Operator1/1
  NoReqV/1 -> Relational Operator6/1
  Switch6/1 -> Unit Delay8/1, [Set3]
  Switch2/1 -> Switch8/1
  Switch12/1 -> Switch11/1
  Switch5/1 -> Switch6/1
  Switch13/1 -> Switch10/1
  [Set] -> Switch5/1
  EEP_Set1/1 -> Switch8/3
  Switch9/1 -> Unit Delay3/1, [Set4]
  EEP_Set7/1 -> Switch11/3
  [Loadbar] -> Switch9/2
  [Set] -> Switch12/1
  Relational Operator/1 -> Unit Delay6/1
  [Set] -> Switch13/1
  [Set] -> Switch3/1
  [Loadbar] -> Switch10/2
  Constant/1 -> Relational Operator/2
  [Loadbar] -> Switch6/2
  [Loadbar] -> Switch11/2
  EEP_Set5/1 -> Switch10/3
  EEP_Set2/1 -> Switch4/3
  [UserNow] -> Relational Operator/1
  Switch4/1 -> Unit Delay2/1, [Set2]
  [Loadbar] -> Switch4/2
  [Set] -> Switch7/1
  EEP_Set4/1 -> Switch9/3
  Switch11/1 -> Unit Delay5/1, [Set7]
  EEP_Set3/1 -> Switch6/3
  [Loadbar] -> Switch8/2
  [UserNow] -> Relational Operator1/1
  Constant1/1 -> Relational Operator1/2
  Relational Operator1/1 -> Unit Delay9/1
  [UserNow] -> Relational Operator2/1
  Constant2/1 -> Relational Operator2/2
  Relational Operator2/1 -> Unit Delay10/1
  [UserNow] -> Relational Operator3/1
  Constant3/1 -> Relational Operator3/2
  Relational Operator3/1 -> Unit Delay11/1
  [UserNow] -> Relational Operator4/1
  Constant4/1 -> Relational Operator4/2
  Relational Operator4/1 -> Unit Delay12/1
  [UserNow] -> Relational Operator5/1
  Constant5/1 -> Relational Operator5/2
  Relational Operator5/1 -> Unit Delay13/1
  Switch3/1 -> Switch4/1
  Detect Change7/1 -> AND11/2
  Switch7/1 -> Switch9/1
  Switch10/1 -> Unit Delay4/1, [Set5]
  Switch8/1 -> Unit Delay7/1, [Set1]
  NOT/1 -> Switch1/2
  [Set] -> Switch2/1
  [Set1] -> Multiport Switch/2
  [Set2] -> Multiport Switch/3
  [Set3] -> Multiport Switch/4
  [Set4] -> Multiport Switch/5
  [Set5] -> Multiport Switch/6
  [Set7] -> Multiport Switch/8
  Default/1 -> Multiport Switch/9, Multiport Switch/7

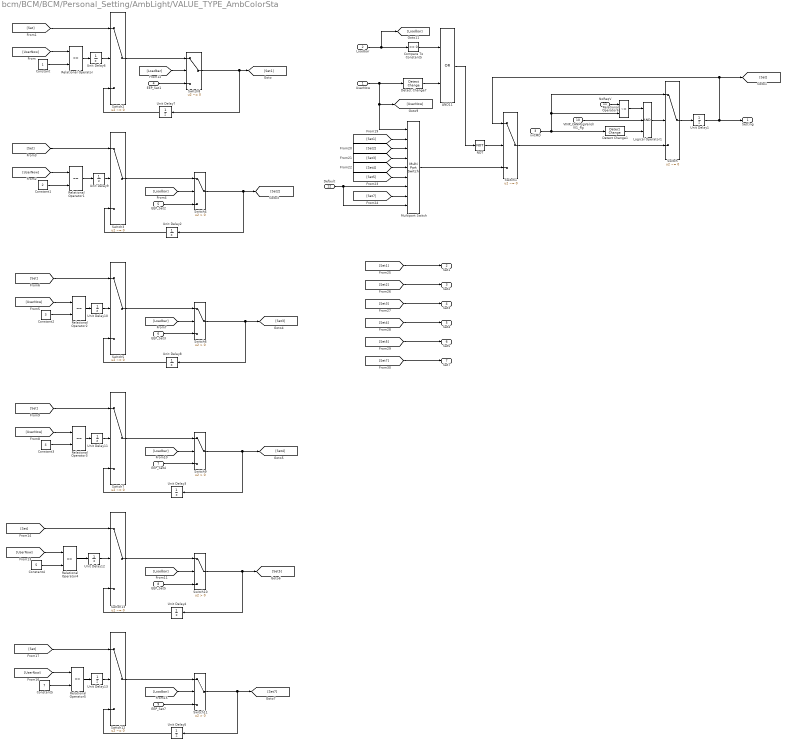
== system bcm/BCM/BCM/Personal_Setting/AmbLight/VALUE_TYPE_AmbColorSta ==
  UserNow : Inport
  Loadbar : Inport  Port=2
  iviCMD : Inport  Port=3
  EEP_Set1 : Inport  Port=4
  EEP_Set2 : Inport  Port=5
  EEP_Set3 : Inport  Port=6
  EEP_Set4 : Inport  Port=7
  EEP_Set5 : Inport  Port=8
  EEP_Set7 : Inport  Port=9
  VINP_CANMsgValidIVI1_flg : Inport  Port=10
  NoReqV : Inport  Port=11
  Default : Inport  Port=12
  AND11 : Logic  Operator=OR  AllPortsSameDT=off  OutDataTypeStr=boolean
  Compare To Constant5 : simulink/Logic and Bit Operations/Compare To Constant  relop===  const=0  OutDataTypeStr=boolean
  Constant : Constant  OutDataTypeStr=uint8
  Constant1 : Constant  Value=2  OutDataTypeStr=uint8
  Constant2 : Constant  Value=3  OutDataTypeStr=uint8
  Constant3 : Constant  Value=4  OutDataTypeStr=uint8
  Constant4 : Constant  Value=5  OutDataTypeStr=uint8
  Constant5 : Constant  Value=7  OutDataTypeStr=uint8
  Detect Change1 : simulink/Logic and Bit Operations/Detect Change  vinit=0  OutDataTypeStr=boolean
  Detect Change7 : simulink/Logic and Bit Operations/Detect Change  vinit=0  OutDataTypeStr=boolean
  Logical Operator1 : Logic  Inputs=3  AllPortsSameDT=off  OutDataTypeStr=boolean
  Multiport Switch : MultiPortSwitch  Inputs=7  DataPortForDefault=Additional data port  DiagnosticForDefault=None
  NOT : Logic  Operator=NOT  IconShape=distinctive  AllPortsSameDT=off  OutDataTypeStr=boolean
  Relational Operator{,1..5} (6 alike) : RelationalOperator  Operator===  OutDataTypeStr=boolean  RndMeth=Simplest
  Relational Operator6 : RelationalOperator  Operator=~=  OutDataTypeStr=boolean  RndMeth=Simplest
  Switch{,1..3,5,7..8,12..13} (9 alike) : Switch  Criteria=u2 ~= 0
  Switch{4,6,9..11} (5 alike) : Switch  Criteria=u2 > Threshold
  Unit Delay{1..13} (13 alike) : UnitDelay  SampleTime=-1  HasFrameUpgradeWarning=on
  Setting : Outport
  Set1 : Outport  Port=2
  Set2 : Outport  Port=3
  Set3 : Outport  Port=4
  Set4 : Outport  Port=5
  Set5 : Outport  Port=6
  Set7 : Outport  Port=7
  wires:
  Default/1 -> Multiport Switch/7, Multiport Switch/9
  [Set7] -> Multiport Switch/8
  [Set5] -> Multiport Switch/6
  [Set4] -> Multiport Switch/5
  [Set3] -> Multiport Switch/4
  [Set2] -> Multiport Switch/3
  [Set1] -> Multiport Switch/2
  [Set] -> Switch2/1
  NOT/1 -> Switch1/2
  Switch8/1 -> [Set1], Unit Delay7/1
  Switch10/1 -> [Set5], Unit Delay4/1
  Switch7/1 -> Switch9/1
  Detect Change7/1 -> AND11/2
  Switch3/1 -> Switch4/1
  Relational Operator5/1 -> Unit Delay13/1
  Constant5/1 -> Relational Operator5/2
  [UserNow] -> Relational Operator5/1
  Relational Operator4/1 -> Unit Delay12/1
  Constant4/1 -> Relational Operator4/2
  [UserNow] -> Relational Operator4/1
  Relational Operator3/1 -> Unit Delay11/1
  Constant3/1 -> Relational Operator3/2
  [UserNow] -> Relational Operator3/1
  Relational Operator2/1 -> Unit Delay10/1
  Constant2/1 -> Relational Operator2/2
  [UserNow] -> Relational Operator2/1
  Relational Operator1/1 -> Unit Delay9/1
  Constant1/1 -> Relational Operator1/2
  [UserNow] -> Relational Operator1/1
  [Loadbar] -> Switch8/2
  EEP_Set3/1 -> Switch6/3
  Switch11/1 -> [Set7], Unit Delay5/1
  EEP_Set4/1 -> Switch9/3
  [Set] -> Switch7/1
  [Loadbar] -> Switch4/2
  Switch4/1 -> [Set2], Unit Delay2/1
  [UserNow] -> Relational Operator/1
  EEP_Set2/1 -> Switch4/3
  EEP_Set5/1 -> Switch10/3
  [Loadbar] -> Switch11/2
  [Loadbar] -> Switch6/2
  Constant/1 -> Relational Operator/2
  [Loadbar] -> Switch10/2
  [Set] -> Switch3/1
  [Set] -> Switch13/1
  Relational Operator/1 -> Unit Delay6/1
  [Set] -> Switch12/1
  [Loadbar] -> Switch9/2
  EEP_Set7/1 -> Switch11/3
  Switch9/1 -> [Set4], Unit Delay3/1
  EEP_Set1/1 -> Switch8/3
  [Set] -> Switch5/1
  Switch13/1 -> Switch10/1
  Switch5/1 -> Switch6/1
  Switch12/1 -> Switch11/1
  Switch2/1 -> Switch8/1
  Switch6/1 -> [Set3], Unit Delay8/1
  NoReqV/1 -> Relational Operator6/1
  Relational Operator6/1 -> Logical Operator1/1
  Detect Change1/1 -> Logical Operator1/3
  iviCMD/1 -> Detect Change1/1, Switch/1, Relational Operator6/2
  Multiport Switch/1 -> Switch1/3
  Logical Operator1/1 -> Switch/2
  Switch1/1 -> Switch/3
  [Set1] -> Set1/1
  [Set2] -> Set2/1
  [Set3] -> Set3/1
  [Set4] -> Set4/1
  [Set5] -> Set5/1
  [Set7] -> Set7/1
  AND11/1 -> NOT/1
  Compare To Constant5/1 -> AND11/1
  UserNow/1 -> Multiport Switch/1, [UserNow], Detect Change7/1
  Loadbar/1 -> [Loadbar], Compare To Constant5/1
  Switch/1 -> Unit Delay1/1
  Unit Delay1/1 -> Switch1/1, [Set], Setting/1
  Unit Delay7/1 -> Switch2/3
  Unit Delay2/1 -> Switch3/3
  Unit Delay8/1 -> Switch5/3
  Unit Delay3/1 -> Switch7/3
  Unit Delay4/1 -> Switch13/3
  Unit Delay5/1 -> Switch12/3
  Unit Delay6/1 -> Switch2/2
  Unit Delay9/1 -> Switch3/2
  Unit Delay10/1 -> Switch5/2
  Unit Delay11/1 -> Switch7/2
  Unit Delay12/1 -> Switch13/2
  Unit Delay13/1 -> Switch12/2
  VINP_CANMsgValidIVI1_flg/1 -> Logical Operator1/2

== stateflow chart bcm/BCM/BCM/AntiTheft/Chart ==
  settings: sampleTime=StepSize
  state AlertTone [parallel]
    settings: executionOrder=11
    state OFF
      en:VBCM_LockAlarm_enum=0;
    state Lock_Success
      en:VBCM_LockAlarm_enum=1;
    (default) -> OFF
    Lock_Success -> OFF : [after(5,tick)]
    AlertTone -> Lock_Success : eLockAlert [IVI_Lock_SoundSW_Sta==1]
  state ATCtrl [parallel]
    settings: executionOrder=5
    state StandBy
      en:ATCtrl=0;
    state Lock
      en:ATCtrl=1;
    note: 350 ms
    state Unlock
      en:ATCtrl=2;
    (default) -> ATCtrl.StandBy
    ATCtrl.StandBy -> ATCtrl.Lock [order 1] : eLampLock
    ATCtrl.Lock -> ATCtrl.StandBy [order 1] : [after(35,tick)]
    ATCtrl.Unlock -> ATCtrl.Lock [order 2] : eLampLock
    ATCtrl.Lock -> ATCtrl.Unlock [order 2] : eLampUnlock
    ATCtrl.StandBy -> ATCtrl.Unlock [order 2] : eLampUnlock
    ATCtrl.Unlock -> ATCtrl.StandBy [order 1] : [after(35,tick)]
  state Main [parallel]
    settings: executionOrder=1
    state sDisarm
      en:AntitheftSta=0;
      fFirst=1;
    state sSecurity
      state sSecurity
        en:
        AntitheftSta=1;
        fFirst=0;
      note: 28 sec
      note: 10 times
      state sAlarm
        en:
        AntitheftSta=3;
        ATAlarm=1;
        Horn.eHornAlarm;
        CountAlarm=CountAlarm+1;
        ex:ATAlarm=0;
      (junction 1705) -> (junction 1971) [order 2] : {Horn.eHornLock;}
      (junction 1705) -> Main.sSecurity.sSecurity [order 1] : [fHornOFF==1||fFirst==1]
          | /{fHornOFF=0;AlertTone.eLockAlert;}
      (junction 1971) -> Main.sSecurity.sSecurity
      Main.sSecurity.sSecurity -> sAlarm : eDoorOpen[CountAlarm<10]
      sAlarm -> Main.sSecurity.sSecurity : [after(2800,tick)]
    note: 1 sec
    state sLockCheck
    (default) -> (junction 2132) : {CountAlarm = VINP_FlashCountAlarm_enum;}
    (junction 2132) -> (junction 2133) [order 1]
    (junction 2133) -> (junction 2135) [order 1]
    (junction 2132) -> sDisarm [order 2]
    (junction 2133) -> Main.sSecurity.sSecurity [order 2] : [VBCM_FlashAntitheft_enum == ENUM_ANTITHEFT_ARM]
    (junction 2135) -> sAlarm : [VBCM_FlashAntitheft_enum == ENUM_ANTITHEFT_ALARM]
    (junction 1713) -> sDisarm : {ATLockCtrl.eActUnlock;Horn.eLockFail;}
    (junction 1703) -> (junction 1713) [order 1] : [!DrLockSta||AllDoorSW||TailgateSW||HoodSW]
    (junction 1703) -> (junction 1705) [order 2] : {CountAlarm=0;}
    (junction 1686) -> (junction 1713) [order 1] : [AllDoorSW||TailgateSW||HoodSW]
    sLockCheck -> (junction 1703) : [after(100,tick)]
    sDisarm -> sDisarm [order 2] : eUnlock{ATCtrl.eLampUnlock;ATLockCtrl.eActUnlock;}
    (junction 1686) -> sLockCheck [order 2] : {ATLockCtrl.eActLock;}
    (junction 1712) -> (junction 1686) : {ATCtrl.eLampLock;}
    sDisarm -> (junction 1712) [order 1] : eLock
    Main.sSecurity -> (junction 1712) [order 2] : eLock
    Main.sSecurity -> sDisarm [order 1] : eUnlock{ATCtrl.eLampUnlock;ATLockCtrl.eActUnlock;}
    Main.sSecurity -> sDisarm [order 3] : eForceDisarm
  state DKCCmd [parallel]
    settings: executionOrder=2
    state WaitForZone
    state Lock
      en:Main.eLock;
    state Unlock
      en:Main.eUnlock;
    state sStandBy
    state Tailgate
      en:DoorSWDetection.TailgateSW.eTailgate;
      PowerTailgate.eTailgateRemote;
    state FindCar
      en:Horn.eHornLock;ATCtrl.eLampUnlock;
    state TailgateLockFail
      en:Horn.eLockFail;Main.eUnlock;
    state TailgateHandle
      en:DoorSWDetection.TailgateSW.eTailgate;
      PowerTailgate.eTailgateHandle;
    state ForceDisarm
      en:Main.eForceDisarm;
    state FindCarMute
      en:ATCtrl.eLampUnlock;
    DKCCmd -> (junction 2148) : [hasChanged(P_CommandtoBCM)]{PcmdBuf=P_CommandtoBCM;}
    (junction 2148) -> DKCCmd.WaitForZone [order 2]
    (junction 2148) -> (junction 2154) [order 1]
    DKCCmd.WaitForZone -> (junction 2154) [order 2]
    (junction 2154) -> (junction 2045) : [VINP_CANMsgValidGWZoneDR1_flg&&VINP_CANMsgValidGWZoneFR1_flg]
    DKCCmd.WaitForZone -> (junction 2151) [order 1] : [after(200,tick)]
    (junction 2151) -> (junction 2045)
    (junction 2045) -> DKCCmd.Lock [order 1] : [VehSpeed<=0&&PcmdBuf==1]
    (junction 2045) -> (junction 2046) [order 2]
    (default) -> DKCCmd.sStandBy : {PcmdBuf=0;}
    (junction 2046) -> DKCCmd.Unlock [order 1] : [VehSpeed<=0&&PcmdBuf==2]
    (junction 2046) -> (junction 2047) [order 2]
    (junction 2047) -> DKCCmd.Tailgate [order 1] : [PcmdBuf==3]
    (junction 2047) -> (junction 2048) [order 2]
    (junction 2048) -> DKCCmd.FindCar [order 1] : [PcmdBuf==4]
    (junction 2048) -> (junction 2049) [order 2]
    (junction 2049) -> TailgateLockFail [order 1] : [PcmdBuf==5]
    (junction 2049) -> (junction 2050) [order 2]
    (junction 2050) -> DKCCmd.TailgateHandle [order 1] : [PcmdBuf==6]
    (junction 2050) -> (junction 2108) [order 2]
    (junction 2108) -> ForceDisarm [order 1] : [PcmdBuf==7]
    (junction 2108) -> (junction 2124) [order 2]
    (junction 2124) -> DKCCmd.sStandBy [order 2]
    (junction 2124) -> DKCCmd.FindCarMute [order 1] : [PcmdBuf==8]
  state DoorSWDetection [parallel]
    settings: executionOrder=4
    state DrDoor [parallel]
      settings: executionOrder=1
      state DrDoorSW_Open
      state DrDoorSW_Close
      (default) -> DrDoorSW_Open
      DrDoorSW_Open -> DrDoorSW_Close : [!DrDoorSW]
      DrDoorSW_Close -> DrDoorSW_Open : [DrDoorSW]/{Main.eDoorOpen;}
    state PsDoor [parallel]
      settings: executionOrder=2
      state PsDoorSW_Open
      state PsDoorSW_Close
      (default) -> PsDoorSW_Open
      PsDoorSW_Open -> PsDoorSW_Close : [!PsDoorSW]
      PsDoorSW_Close -> PsDoorSW_Open : [PsDoorSW]/{Main.eDoorOpen;}
    state RLDoor [parallel]
      settings: executionOrder=3
      state RLDoorSW_Open
      state RLDoorSW_Close
      (default) -> RLDoorSW_Open
      RLDoorSW_Open -> RLDoorSW_Close : [!RLDoorSW]
      RLDoorSW_Close -> RLDoorSW_Open : [RLDoorSW]/{Main.eDoorOpen;}
    state RRDoor [parallel]
      settings: executionOrder=4
      state RRDoorSW_Open
      state RRDoorSW_Close
      (default) -> RRDoorSW_Open
      RRDoorSW_Open -> RRDoorSW_Close : [!RRDoorSW]
      RRDoorSW_Close -> RRDoorSW_Open : [RRDoorSW]/{Main.eDoorOpen;}
    state HoodSW [parallel]
      settings: executionOrder=5
      state HoodSW_Open
      state HoodSW_Close
      (default) -> HoodSW_Open
      HoodSW_Open -> HoodSW_Close : [!HoodSW]
      HoodSW_Close -> HoodSW_Open : [HoodSW]/{Main.eDoorOpen;}
    state TailgateSW [parallel]
      settings: executionOrder=6
      state TailgateSW_Open
      state TailgateSW_Close
      state sRemote
      state Ignore
      (default) -> TailgateSW_Open
      TailgateSW_Open -> TailgateSW_Close : [!TailgateSW]
      TailgateSW_Close -> TailgateSW_Open [order 1] : [TailgateSW]/{Main.eDoorOpen;}
      TailgateSW_Close -> sRemote [order 2] : eTailgate
      (junction 1886) -> TailgateSW_Close [order 2] : [after(1500,tick)]
      Ignore -> TailgateSW_Close : [!TailgateSW]
      sRemote -> (junction 1886)
      (junction 1886) -> Ignore [order 1] : [TailgateSW]
    note: 15 sec
  state Horn [parallel]
    settings: executionOrder=3
    state sStandBy
      en:HornCtrl=0;
    note: 250 ms
    state sAlarm2
      en:HornCtrl=0;
    state sAlarm1
      en:HornCtrl=1;
    state sLock
      en:HornCtrl=1;
    state sKeyIN1
      en:HornCtrl=1;
    state sKeyIN2
      en:HornCtrl=0;
    state sLockFail1
      en:HornCtrl=1;
    state sLockFail2
      en:HornCtrl=0;
    state sLockFail3
      en:HornCtrl=1;
    (default) -> Horn.sStandBy
    (junction 1821) -> Horn.sStandBy
    sAlarm1 -> sAlarm2 : [after(25,tick)]
    sAlarm2 -> (junction 1821) [order 1] : [ATAlarm==0]
    Horn -> sAlarm1 [order 1] : eHornAlarm
    (junction 1827) -> (junction 1821)
    sAlarm2 -> sAlarm1 [order 2] : [after(25,tick)]
    sLock -> (junction 1827) : [after(3,tick)]
    (junction 2026) -> (junction 1827)
    Horn -> sLock [order 2] : eHornLock
    sKeyIN2 -> sLock : [after(5,tick)]
    Horn -> sKeyIN1 [order 3] : eKeyIN
    sKeyIN1 -> sKeyIN2 : [after(3,tick)]
    Horn -> sLockFail1 [order 4] : eLockFail
    sLockFail1 -> sLockFail2 : [after(10,tick)]
    sLockFail2 -> sLockFail3 : [after(30,tick)]
    sLockFail3 -> (junction 2026) : [after(10,tick)]
  state ATLockCtrl [parallel]
    settings: executionOrder=6
    state Lock
      en:ATLockCtrl=1;
    state StandBy
      en:ATLockCtrl=0;
    note: 350 ms
    state Unlock
      en:ATLockCtrl=2;
    (default) -> ATLockCtrl.StandBy
    ATLockCtrl.StandBy -> ATLockCtrl.Lock [order 1] : eActLock
    ATLockCtrl.Lock -> ATLockCtrl.StandBy : [after(35,tick)]
    ATLockCtrl.Unlock -> ATLockCtrl.Lock [order 2] : eActLock
    ATLockCtrl.StandBy -> ATLockCtrl.Unlock [order 2] : eActUnlock
    ATLockCtrl.Unlock -> ATLockCtrl.StandBy [order 1] : [after(35,tick)]
  state VIGCommand [parallel]
    settings: executionOrder=7
    state WaitForZone
    state StandBy
    state Lock
      en:Main.eLock;
    state Unlock
      en:Main.eUnlock;
    state FindCar
      en:Horn.eHornLock;ATCtrl.eLampUnlock;
    state FindCarMute
      en:ATCtrl.eLampUnlock;
    state Tailgate
      en:DoorSWDetection.TailgateSW.eTailgate;
      PowerTailgate.eTailgateRemote;
    state TailgateReject
      en:PowerTailgate.eTailgateReject;
    (default) -> VIGCommand.WaitForZone
    VIGCommand.WaitForZone -> VIGCommand.StandBy : [VINP_CANMsgValidGWZoneDR1_flg&&VINP_CANMsgValidGWZoneFR1_flg]
    VIGCommand.StandBy -> VIGCommand.Lock [order 1] : [VehSpeed<=0&&(VIG_Cmd==1||VIG_Cmd==5)]
    VIGCommand.Lock -> VIGCommand.StandBy : [VIG_Cmd==0]
    (junction 1941) -> VIGCommand.Lock [order 1] : [AntitheftSta==0||AntitheftSta==2]/{fHornOFF=1;}
    VIGCommand.StandBy -> (junction 1941) [order 6] : [VehSpeed<=0&&VIG_Cmd==7]
    (junction 1941) -> VIGCommand.Unlock [order 2] : [fVIGHandle==0]
    VIGCommand.StandBy -> VIGCommand.Unlock [order 2] : [VehSpeed<=0&&(VIG_Cmd==2||VIG_Cmd==6)]
    VIGCommand.Unlock -> VIGCommand.StandBy : [VIG_Cmd==0]
    VIGCommand.StandBy -> VIGCommand.FindCar [order 3] : [VIG_Cmd==3]
    VIGCommand.FindCar -> VIGCommand.StandBy : [VIG_Cmd==0]
    VIGCommand.StandBy -> VIGCommand.FindCarMute [order 5] : [VIG_Cmd==8]
    VIGCommand.FindCarMute -> VIGCommand.StandBy : [VIG_Cmd==0]
    VIGCommand.Tailgate -> VIGCommand.StandBy : [VIG_Cmd==0]
    (junction 2118) -> VIGCommand.Tailgate
    (junction 2116) -> (junction 2118) [order 2]
    VIGCommand.StandBy -> (junction 2116) [order 4] : [VIG_Cmd==4]
    (junction 2116) -> TailgateReject [order 1] : [PwrSta==5]
    TailgateReject -> VIGCommand.StandBy : [VIG_Cmd==0]
  state PowerTailgate [parallel]
    settings: executionOrder=9
    state StandBy
      en:TailgateRemote=0;
    state TailgateRemote
      en:TailgateRemote=1;
    note: 200 ms
    state TailgateHandle
      en:TailgateRemote=2;
    note: 200 ms
    state TailgateHandle1
      en:TailgateRemote=3;
    (default) -> PowerTailgate.StandBy
    PowerTailgate.StandBy -> TailgateRemote [order 1] : eTailgateRemote
    TailgateRemote -> PowerTailgate.StandBy : [after(20,tick)]
    PowerTailgate.StandBy -> PowerTailgate.TailgateHandle [order 2] : eTailgateHandle
    PowerTailgate.TailgateHandle -> PowerTailgate.StandBy : [after(20,tick)]
    PowerTailgate.StandBy -> TailgateHandle1 [order 3] : eTailgateReject
    TailgateHandle1 -> PowerTailgate.StandBy : [after(20,tick)]
  state AGSTailgateOpen [parallel]
    settings: executionOrder=8
    state sStandBy
    state Tailgate
      en:DoorSWDetection.TailgateSW.eTailgate;
      PowerTailgate.eTailgateRemote;
    (default) -> AGSTailgateOpen.sStandBy
    AGSTailgateOpen.sStandBy -> AGSTailgateOpen.Tailgate : [APSOpenPTG==1&&TailgateSW==0]
    AGSTailgateOpen.Tailgate -> AGSTailgateOpen.sStandBy : [APSOpenPTG==0]
  state AntitheftSeat [parallel]
    settings: executionOrder=10
    state StandBy
      en:AntitheftSeatFlod=0;
    state Lock_Check
      en:AntitheftSeatFlod=0;
    state Flod
      en:AntitheftSeatFlod=1;
    note: 200 ms
    (default) -> AntitheftSeat.StandBy
    AntitheftSeat.StandBy -> Lock_Check : [fHornOFF==1]
    Lock_Check -> Flod : [fHornOFF==0]
    Flod -> Lock_Check [order 2] : [fHornOFF==1]
    Flod -> AntitheftSeat.StandBy [order 1] : [after(20,tick)]
  data: P_CommandtoBCM input uint8 [0..11]; PwrSta input uint8 [0..5]; ATCtrl output uint8; ATLockCtrl output uint8; AllDoorSW input boolean [0..1]; HoodSW input boolean; TailgateSW input boolean; DrDoorSW input boolean; PsDoorSW input boolean; RLDoorSW input boolean; RRDoorSW input boolean; DrLockSta input boolean; ATAlarm output boolean; AntitheftSta output uint8; TailgateRemote output uint8; HornCtrl output boolean; VIG_Cmd input uint8 [0..7]; VehSpeed input single [0..1]; fVIGHandle input boolean; VBCM_FlashAntitheft_enum input uint8; fFirst local boolean; fHornOFF local boolean; AntitheftSeatFlod output boolean; APSOpenPTG input boolean; ENUM_ANTITHEFT_ALARM parameter uint8; ENUM_ANTITHEFT_ARM parameter uint8; VINP_FlashCountAlarm_enum input uint8; VINP_CANMsgValidGWZoneDR1_flg input boolean; VINP_CANMsgValidGWZoneFR1_flg input boolean; PcmdBuf local uint8; CountAlarm output uint8; IVI_Lock_SoundSW_Sta input boolean; VBCM_LockAlarm_enum output uint8
  data PwrSta settings: description=Min=0, Max=2047, Engineering Unit = km/h, Offset=0 km/h, Resolution= 0.125 km/h per bit, >2047 = Invalid (bit 12 = 1)
  events: eLockAlert local FUNCTION_CALL_EVENT; eLampLock local FUNCTION_CALL_EVENT; eLampUnlock local FUNCTION_CALL_EVENT; eLock local FUNCTION_CALL_EVENT; eUnlock local FUNCTION_CALL_EVENT; eDoorOpen local FUNCTION_CALL_EVENT; eForceDisarm local FUNCTION_CALL_EVENT; eTailgate local FUNCTION_CALL_EVENT; eHornAlarm local FUNCTION_CALL_EVENT; eHornLock local FUNCTION_CALL_EVENT; eKeyIN local FUNCTION_CALL_EVENT; eLockFail local FUNCTION_CALL_EVENT; eActLock local FUNCTION_CALL_EVENT; eActUnlock local FUNCTION_CALL_EVENT; eTailgateRemote local FUNCTION_CALL_EVENT; eTailgateHandle local FUNCTION_CALL_EVENT; eTailgateReject local FUNCTION_CALL_EVENT
